simulink library "mylib"  (R2020a)
settings: Solver=VariableStepAuto  StartTime=0.0  StopTime=10.0  RelTol=1e-3
undefined symbols (not defined in the file): d_du_max_pu, dir_to_bus1, dir_to_bus_0L, dir_to_bus_2, dir_to_line1, dir_to_line_0L, dir_to_line_2, du_max_pu, du_ph_max_pu, Fi_0, Fi_T_H, Fi_T_L, Fi_T_M, I0_calc_0L, I0_comp_H, I0_comp_L, I0_comp_M, I0_max_0L, I2_max_2, I_diff1, I_diff2, I_diff3, I_diff4, I_diff5, I_diff_to, I_hight_CT1_G, I_hight_CT2_G, I_low_CT1, I_low_CT2, I_max1, I_max2, I_max3, I_max4, I_max5, I_min_sec_CT1, I_min_sec_CT2, I_unb, Iph_max_0L, Iph_max_2, jmp_in_zone, jmp_in_zone_0L, jmp_in_zone_2, K_dop, max_min1, only_K1_0L, only_K1_2, only_K2_0L, only_K2_2, only_K3_0L, only_K3_2, P_ctl_0, PQ_Fi_ctl_0, Q_ctl_0, S_set_0, set, set1, T_fast, T_I_ctl, T_off, T_on ... (+15)
libraries: $bdroot x184, powerlib_meascontrol x97
(part 3 of 14)

== system mylib/relative ==
  a_re : Inport
  a_im : Inport  Port=2
  1 : Sum  Inputs=+-
  10 : Product  Inputs=*/  RndMeth=Zero  SaturateOnIntegerOverflow=on
  2 : Sum  Inputs=+-
  3 : MinMax  Function=max  Inputs=2
  4 : RelationalOperator  Operator===  OutDataTypeStr=boolean  RndMeth=Simplest
  5 : RelationalOperator  Operator===  OutDataTypeStr=boolean  RndMeth=Simplest
  6 : Switch  Criteria=u2 > Threshold
  7 : RelationalOperator  Operator===  OutDataTypeStr=boolean  RndMeth=Simplest
  8 : Constant  Value=0
  9 : Constant  Value=0.0000001
  fifo1 : Subsystem
  fifo2 : Subsystem
  module1 : Subsystem
  module2 : Subsystem
  module3 : Subsystem
  Y : Outport
  Y_abs : Outport  Port=2
  up : Outport  Port=3
  down : Outport  Port=4
  wires:
  fifo1/1(y0) -> module2/1(Re), 1/1
  fifo1/5(y4) -> module3/1(Re), 1/2
  fifo2/1(y0) -> module2/2(Im), 2/1
  fifo2/5(y4) -> module3/2(Im), 2/2
  1/1 -> module1/1(Re)
  2/1 -> module1/2(Im)
  3/1 -> 5/1, 7/1, 6/3, 4/2
  module2/1(Module) -> 3/1, 4/1
  module3/1(Module) -> 3/2, 5/2
  7/1 -> 6/2
  8/1 -> 7/2
  9/1 -> 6/1
  5/1 -> down/1
  4/1 -> up/1
  module1/1(Module) -> 10/1, Y_abs/1
  6/1 -> 10/2
  10/1 -> Y/1
  a_im/1 -> fifo2/1(y)
  a_re/1 -> fifo1/1(y)

== system mylib/simpcomp ==
  FAre : Inport
  FAim : Inport  Port=2
  FBre : Inport  Port=3
  FBim : Inport  Port=4
  FCre : Inport  Port=5
  FCim : Inport  Port=6
  1 : Constant  Value=-0.5
  {3..5,9..11,18..23} (12 alike) : Sum
  {2,12..16} (6 alike) : Product
  17 : Constant  Value=0.33333333333
  6 : Constant  Value=0.8660254037844386
  7 : Constant  Value=-0.8660254037844386
  orto_MUL_orto : Subsystem
  orto_MUL_orto1 : Subsystem
  orto_MUL_orto2 : Subsystem
  orto_MUL_orto3 : Subsystem
  F0re : Outport
  F0im : Outport  Port=2
  F1re : Outport  Port=3
  F1im : Outport  Port=4
  F2re : Outport  Port=5
  F2im : Outport  Port=6
  wires:
  1/1 -> orto_MUL_orto1/3(F2re), orto_MUL_orto/3(F2re), orto_MUL_orto2/3(F2re), orto_MUL_orto3/3(F2re)
  6/1 -> orto_MUL_orto2/4(F2im), orto_MUL_orto/4(F2im)
  7/1 -> orto_MUL_orto3/4(F2im), orto_MUL_orto1/4(F2im)
  15/1 -> F2im/1
  14/1 -> F2re/1
  16/1 -> F1im/1
  13/1 -> F1re/1
  2/1 -> F0re/1
  12/1 -> F0im/1
  5/1 -> 2/1
  3/1 -> 12/1
  4/1 -> 13/1
  11/1 -> 16/1
  9/1 -> 14/1
  10/1 -> 15/1
  20/1 -> 10/2
  23/1 -> 9/2
  21/1 -> 11/2
  22/1 -> 4/2
  18/1 -> 3/1
  19/1 -> 5/1
  FAim/1 -> 10/1, 3/2, 11/1
  FAre/1 -> 9/1, 5/2, 4/1
  orto_MUL_orto2/2(Fim) -> 20/2
  orto_MUL_orto1/2(Fim) -> 20/1
  orto_MUL_orto2/1(Fre) -> 23/2
  orto_MUL_orto1/1(Fre) -> 23/1
  orto_MUL_orto3/2(Fim) -> 21/2
  orto_MUL_orto/2(Fim) -> 21/1
  orto_MUL_orto3/1(Fre) -> 22/2
  orto_MUL_orto/1(Fre) -> 22/1
  FBre/1 -> orto_MUL_orto1/1(F1re), 19/1, orto_MUL_orto/1(F1re)
  FBim/1 -> orto_MUL_orto1/2(F1im), 18/1, orto_MUL_orto/2(F1im)
  FCim/1 -> 18/2, orto_MUL_orto2/2(F1im), orto_MUL_orto3/2(F1im)
  FCre/1 -> orto_MUL_orto3/1(F1re), 19/2, orto_MUL_orto2/1(F1re)
  17/1 -> 15/2, 14/2, 13/2, 12/2, 2/2, 16/2

== system mylib/st_inverse ==
  block1 : Inport
  block2 : Inport  Port=2
  block3 : Inport  Port=3
  block4 : Inport  Port=4
  in : Inport  Port=5
  alt_in : Inport  Port=6
  jmp : Inport  Port=7
  I_re : Inport  Port=8
  I_im : Inport  Port=9
  1 : Logic  Operator=OR  Inputs=4  AllPortsSameDT=off  OutDataTypeStr=boolean
  Cast To Double : DataTypeConversion  OutDataTypeStr=double
  Constant4 : Constant  Value=jmp_in_zone
  Inverse time-delay : Subsystem  mask{Itd=[14.7, 1, 1], IEC=[4, 3, 9, 0.05], IEC_idr=[4, 7, 2], ANSI=[7, 3, 7, 9.3, 0.08], ANSI_idr=[7, 5, 4.1, 0]}
      mask prompts: Itd "Itd [Ip, Type_ITD, IDR]"; IEC "IEC [IEC_N, ku_IEC, au_IEC, Tb]"; IEC_idr "IEC_idr [IEC_N_idr, ku_IEC_idr, au_IEC_idr]"; ANSI "ANSI [ANSI_N, Au_ANSI, Bu_ANSI, Cu_ANSI, D]"; ANSI_idr "ANSI_idr [ANSI_N_idr, Au_ANSI_idr, Bu_ANSI_idr, Cu_ANSI_idr]"
      mask init: same as mylib/Inverse time-delay
      mask DialogControl Control2 Prompt: Inverse time-delay
      mask DialogControl Control3 Prompt: IEC
      mask DialogControl Control4 Prompt: IEC_idr
      mask DialogControl Control5 Prompt: ANSI
      mask DialogControl Control6 Prompt: ANSI_idr
  Logical Operator14 : Logic  Operator=OR  AllPortsSameDT=off  OutDataTypeStr=boolean
  Logical Operator2 : Logic  AllPortsSameDT=off  OutDataTypeStr=boolean
  Logical Operator3 : Logic  Operator=NOT  AllPortsSameDT=off  OutDataTypeStr=boolean
  Logical Operator8 : Logic  AllPortsSameDT=off  OutDataTypeStr=boolean
  ORTOTOMODULE : $bdroot/ORTOTOMODULE  SystemSampleTime=-1  Latency=0  AutoFrameSizeCalculation=off
  R_TRIG : $bdroot/R_TRIG  SystemSampleTime=-1  Latency=0  AutoFrameSizeCalculation=off
  Variable Transport Delay : VariableTransportDelay  VariableDelayType=Variable transport delay  MaximumDelay=100
  in_1 : Subsystem  mask{in_jmp=[T_reset]}
      mask prompts: in_jmp "in_jmp[T_reset]"
  out_a : $bdroot/out3  out=[T_out]
  avar : Outport
  Y : Outport  Port=2
  fast : Outport  Port=3
  wires:
  block1/1 -> 1/1
  block2/1 -> 1/2
  block3/1 -> 1/3
  block4/1 -> 1/4
  in/1 -> Logical Operator8/2, in_1/2(in)
  R_TRIG/1 -> avar/1
  Constant4/1 -> in_1/1(jmp_in_zone)
  jmp/1 -> in_1/3(jmp)
  Logical Operator3/1 -> Logical Operator2/1
  in_1/1(Y) -> Logical Operator2/2  "Ya"
  1/1 -> Logical Operator3/1
  out_a/1 -> R_TRIG/1, Y/1  "Y_c"
  Logical Operator8/1 -> out_a/1
  Variable Transport Delay/1 -> Logical Operator8/1
  Logical Operator2/1 -> fast/1, Logical Operator14/1
  alt_in/1 -> Logical Operator14/2
  I_im/1 -> ORTOTOMODULE/2
  I_re/1 -> ORTOTOMODULE/1
  ORTOTOMODULE/1 -> Inverse time-delay/1(I)
  Inverse time-delay/1(tp) -> Variable Transport Delay/2
  Inverse time-delay/2(td) -> in_1/4(T_reset)
  Logical Operator14/1 -> Cast To Double/1
  Cast To Double/1 -> Variable Transport Delay/1

== system mylib/tzop_st_v1 ==
  fast1_time : Inport
  fast2_time : Inport  Port=2
  fast3_time : Inport  Port=3
  fast4_time : Inport  Port=4
  fast1_zero : Inport  Port=5
  fast2_zero : Inport  Port=6
  fast3_zero : Inport  Port=7
  fast4_zero : Inport  Port=8
  block1 : Inport  Port=9
  block2 : Inport  Port=10
  block3 : Inport  Port=11
  block4 : Inport  Port=12
  no_dir1 : Inport  Port=13
  no_dir2 : Inport  Port=14
  no_dir3 : Inport  Port=15
  no_dir4 : Inport  Port=16
  dir_to_line : Inport  Port=17
  Ia_re : Inport  Port=18
  Ia_im : Inport  Port=19
  Ib_re : Inport  Port=20
  Ib_im : Inport  Port=21
  Ic_re : Inport  Port=22
  Ic_im : Inport  Port=23
  jmp_a : Inport  Port=24
  jmp_b : Inport  Port=25
  jmp_c : Inport  Port=26
  {1..3,33} (4 alike) : Logic  Operator=OR  Inputs=4  AllPortsSameDT=off  OutDataTypeStr=boolean
  200_det18_ph : Subsystem  mask{det=[0, Iph_max, 0, 0]}
      mask prompts: det "det [max_min, set, dir_to_line, dir_to_bus]"
      mask init:
      | max_min = det(1);
      | set = det(2);
      | dir_to_line = det(3);
      | dir_to_bus = det(4);
  218_det18 : Subsystem  mask{det=[0, I2_max, dir_to_line, dir_to_bus]}
      mask prompts: det "det [max_min, set, dir_to_line, dir_to_bus]"
      mask init:
      | max_min = det(1);
      | set = det(2);
      | dir_to_line = det(3);
      | dir_to_bus = det(4);
  230_st18_ph : Subsystem  AncestorBlock=mylib/230_st18_ph  mask{st18_ph=[only_K1, only_K2, only_K3, jmp_in_zone, T_reset, T_fast, T_st, T_out]}
      mask prompts: st18_ph "st18_ph [only_K1, only_K2, only_K3, jmp_in_zone, T_reset, T_fast, T_st, T_out]"
      mask init:
      | only_K1 = st18_ph(1);
      | only_K2 = st18_ph(2); 
      | only_K3 = st18_ph(3); 
      | jmp_in_zone = st18_ph(4);
      | T_reset = st18_ph(5);
      | T_fast = st18_ph(6); 
      | T_st = st18_ph(7); 
      | T_out = st18_ph(8);
  Constant : Constant
  Constant10 : Constant  Value=0
  Constant11 : Constant  Value=0
  Constant12 : Constant
  Constant13 : Constant  Value=0
  simpcomp : $bdroot/simpcomp  SystemSampleTime=-1  Latency=0  AutoFrameSizeCalculation=off
  avar : Outport
  avar1 : Outport  Port=2
  Y : Outport  Port=3
  Y_a : Outport  Port=4
  Y_b : Outport  Port=5
  Y_c : Outport  Port=6
  fast : Outport  Port=7
  fast_a : Outport  Port=8
  fast_b : Outport  Port=9
  fast_c : Outport  Port=10
  wires:
  Constant13/1 -> 200_det18_ph/2(start2), 200_det18_ph/3(start3), 200_det18_ph/4(start4), 200_det18_ph/6(block2), 200_det18_ph/7(block3), 200_det18_ph/11(no_dir3), 200_det18_ph/12(no_dir4), 200_det18_ph/13(block_a), 200_det18_ph/14(block_b), 200_det18_ph/15(block_c), 200_det18_ph/22(dir_to_line_a), 200_det18_ph/23(dir_to_line_b), 200_det18_ph/24(dir_to_line_c), 200_det18_ph/10(no_dir2), 200_det18_ph/8(block4)
  Constant12/1 -> 200_det18_ph/9(no_dir1)
  1/1 -> 230_st18_ph/3(fast1_zero)
  33/1 -> 230_st18_ph/1(fast1_time)
  218_det18/2(Y) -> 200_det18_ph/1(start1)
  jmp_c/1 -> 230_st18_ph/17(jmp_c)
  jmp_b/1 -> 230_st18_ph/16(jmp_b)
  jmp_a/1 -> 230_st18_ph/15(jmp_a)
  Constant11/1 -> 230_st18_ph/2(fast2_time), 230_st18_ph/4(fast2_zero), 230_st18_ph/6(block2), 230_st18_ph/7(block3), 230_st18_ph/8(block4), 230_st18_ph/12(alt_in_a), 230_st18_ph/13(alt_in_b), 230_st18_ph/14(alt_in_c)
  200_det18_ph/5(Y_c) -> 230_st18_ph/11(in_c)
  200_det18_ph/4(Y_b) -> 230_st18_ph/10(in_b)
  200_det18_ph/3(Y_a) -> 230_st18_ph/9(in_a)
  230_st18_ph/6(fast) -> fast/1
  230_st18_ph/7(fast_a) -> fast_a/1
  230_st18_ph/8(fast_b) -> fast_b/1
  230_st18_ph/9(fast_c) -> fast_c/1
  230_st18_ph/5(Y_c) -> Y_c/1
  230_st18_ph/4(Y_b) -> Y_b/1
  230_st18_ph/3(Y_a) -> Y_a/1
  230_st18_ph/2(Y) -> Y/1
  230_st18_ph/1(avar) -> avar1/1
  2/1 -> 230_st18_ph/5(block1), 218_det18/5(block1)
  3/1 -> 218_det18/9(no_dir1)
  Constant10/1 -> 218_det18/2(start2), 218_det18/3(start3), 218_det18/4(start4), 218_det18/6(block2), 218_det18/7(block3), 218_det18/8(block4), 218_det18/10(no_dir2), 218_det18/11(no_dir3), 218_det18/12(no_dir4)
  Constant/1 -> 218_det18/1(start1)
  dir_to_line/1 -> 218_det18/15(dir_to_line)
  simpcomp/6 -> 218_det18/14(in_im)
  simpcomp/5 -> 218_det18/13(in_re)
  Ic_im/1 -> simpcomp/6, 200_det18_ph/21(in_c_im)
  Ic_re/1 -> simpcomp/5, 200_det18_ph/20(in_c_re)
  Ib_im/1 -> simpcomp/4, 200_det18_ph/19(in_b_im)
  Ib_re/1 -> simpcomp/3, 200_det18_ph/18(in_b_re)
  Ia_im/1 -> simpcomp/2, 200_det18_ph/17(in_a_im)
  Ia_re/1 -> simpcomp/1, 200_det18_ph/16(in_a_re)
  no_dir1/1 -> 3/1
  no_dir3/1 -> 3/3
  no_dir4/1 -> 3/4
  no_dir2/1 -> 3/2
  fast1_time/1 -> 33/1
  fast2_time/1 -> 33/2
  fast3_time/1 -> 33/3
  fast4_time/1 -> 33/4
  fast1_zero/1 -> 1/1
  fast2_zero/1 -> 1/2
  fast3_zero/1 -> 1/3
  fast4_zero/1 -> 1/4
  block1/1 -> 2/1
  block2/1 -> 2/2
  block3/1 -> 2/3
  block4/1 -> 2/4
  218_det18/1(avar) -> avar/1

== system mylib/vect_to_pu ==
  In_re : Inport
  In_im : Inport  Port=2
  1 : Product  Inputs=**
  2 : Sum
  3 : Product  Inputs=*/
  4 : Sqrt  SaturateOnIntegerOverflow=on
  5 : Product  Inputs=**
  6 : Product  Inputs=*/
  out_re : Outport
  out_im : Outport  Port=2
  wires:
  5/1 -> 2/2
  1/1 -> 2/1
  2/1 -> 4/1
  6/1 -> out_re/1
  In_re/1 -> 6/1, 1/2, 1/1
  In_im/1 -> 3/1, 5/2, 5/1
  3/1 -> out_im/1
  4/1 -> 3/2, 6/2

== system mylib/205_st18/Subsystem ==
  T_fast_time : Inport
  T_fast_zero : Inport  Port=2
  "In1 " : Inport  Port=3
  5 : Switch  Criteria=u2 > Threshold
  7 : Switch  Criteria=u2 > Threshold
  T3 : powerlib_meascontrol/Logic/On Delay  DelayType=On delay  delay=T_st  ic=0  Ts=0
  T6 : powerlib_meascontrol/Logic/On Delay  DelayType=On delay  delay=T_fast  ic=0  Ts=0
  T7 : powerlib_meascontrol/Logic/On Delay  DelayType=Off delay  delay=T_fast  ic=0  Ts=0
  Out1 : Outport
  wires:
  "In1 "/1 -> T6/1, 5/1, T3/1
  T7/1 -> 7/2
  T_fast_time/1 -> T7/1
  T6/1 -> 7/1
  T3/1 -> 7/3
  T_fast_zero/1 -> 5/2
  7/1 -> 5/3
  5/1 -> Out1/1

== system mylib/205_st18/in_1 ==
  jmp_in_zone : Inport
  in : Inport  Port=2
  jmp : Inport  Port=3
  1 : Switch  Criteria=u2 > Threshold
  10 : Logic  AllPortsSameDT=off  OutDataTypeStr=boolean
  11 : Logic  Operator=NOT  AllPortsSameDT=off  OutDataTypeStr=boolean
  12 : Memory
  3 : Logic  AllPortsSameDT=off  OutDataTypeStr=boolean
  RS : $bdroot/RS  SystemSampleTime=-1  Latency=0  AutoFrameSizeCalculation=off
  R_TRIG : $bdroot/R_TRIG  SystemSampleTime=-1  Latency=0  AutoFrameSizeCalculation=off
  T1 : powerlib_meascontrol/Logic/On Delay  DelayType=Off delay  delay=T_reset  ic=0  Ts=0
  T2 : powerlib_meascontrol/Logic/On Delay  DelayType=On delay  delay=T_reset  ic=0  Ts=0
  Y : Outport
  wires:
  RS/1 -> 12/1, Y/1
  in/1 -> 11/1, R_TRIG/1, 1/3
  R_TRIG/1 -> 1/1
  jmp_in_zone/1 -> 1/2
  11/1 -> 10/2
  10/1 -> T2/1
  T1/1 -> 3/2
  1/1 -> 3/1
  jmp/1 -> T1/1
  12/1 -> 10/1
  T2/1 -> RS/2
  3/1 -> RS/1

== system mylib/219_onm_v1/onm_fi_v1 ==
  U_re : Inport
  U_im : Inport  Port=2
  I_re : Inport  Port=3
  I_im : Inport  Port=4
  Constant : Constant  Value=-1
  Constant1 : Constant  Value=-1
  Constant2 : Constant  Value=S_set
  Constant3 : Constant  Value=Fi
  Constant4 : Constant  Value=0.0174532925
  Constant5 : Constant  Value=-1
  Cos : Trigonometry  Operator=cos
  Divide{,1..3} (4 alike) : Product  Inputs=**
  Logical Operator : Logic  Operator=NOT  AllPortsSameDT=off  OutDataTypeStr=boolean
  Logical Operator1 : Logic  Operator=NOT  AllPortsSameDT=off  OutDataTypeStr=boolean
  Relational Operator : RelationalOperator  Operator=<  OutDataTypeStr=boolean  RndMeth=Simplest
  Relational Operator1 : RelationalOperator  Operator=>  OutDataTypeStr=boolean  RndMeth=Simplest
  S_calc : $bdroot/orto_MUL_orto  SystemSampleTime=-1  Latency=0  AutoFrameSizeCalculation=off
  S_protection_calc : $bdroot/orto_MUL_orto  SystemSampleTime=-1  Latency=0  AutoFrameSizeCalculation=off
  Sin : Trigonometry
  Switch : Switch  Criteria=u2 > Threshold
  Y : Outport
  wires:
  Relational Operator1/1 -> Logical Operator/1, Switch/3
  Logical Operator/1 -> Switch/2
  Logical Operator1/1 -> Switch/1
  Switch/1 -> Y/1
  Relational Operator/1 -> Logical Operator1/1
  S_protection_calc/1 -> Relational Operator/1, Relational Operator1/1
  Constant2/1 -> Divide3/1, Relational Operator1/2
  Constant5/1 -> Divide3/2
  Divide3/1 -> Relational Operator/2
  Divide1/1 -> S_protection_calc/4
  Cos/1 -> S_protection_calc/3
  Constant3/1 -> Divide2/1
  Constant4/1 -> Divide2/2
  Divide2/1 -> Cos/1, Sin/1
  Constant1/1 -> Divide1/2
  Sin/1 -> Divide1/1
  S_calc/2 -> S_protection_calc/2
  S_calc/1 -> S_protection_calc/1
  Constant/1 -> Divide/2
  Divide/1 -> S_calc/4
  I_im/1 -> Divide/1
  I_re/1 -> S_calc/3
  U_re/1 -> S_calc/1
  U_im/1 -> S_calc/2

== system mylib/219_onm_v1/pq_dir_v1 ==
  U_re : Inport
  U_im : Inport  Port=2
  I_re : Inport  Port=3
  I_im : Inport  Port=4
  max_comp : Inport  Port=5
  Add : Sum
  Constant : Constant  Value=-1
  Constant1 : Constant  Value=-1
  Constant2 : Constant  Value=P_ctl
  Constant3 : Constant  Value=Q_ctl
  Constant4 : Constant  Value=0
  Constant5 : Constant  Value=0
  Divide{,1..3} (4 alike) : Product  Inputs=**
  Logical Operator : Logic  Operator=NOT  AllPortsSameDT=off  OutDataTypeStr=boolean
  Logical Operator1 : Logic  AllPortsSameDT=off  OutDataTypeStr=boolean
  Logical Operator2 : Logic  AllPortsSameDT=off  OutDataTypeStr=boolean
  Logical Operator3 : Logic  Operator=OR  AllPortsSameDT=off  OutDataTypeStr=boolean
  Relational Operator1 : RelationalOperator  Operator=>  OutDataTypeStr=boolean  RndMeth=Simplest
  Relational Operator2 : RelationalOperator  Operator=>  OutDataTypeStr=boolean  RndMeth=Simplest
  Relational Operator3 : RelationalOperator  Operator=>  OutDataTypeStr=boolean  RndMeth=Simplest
  S_calc : $bdroot/orto_MUL_orto  SystemSampleTime=-1  Latency=0  AutoFrameSizeCalculation=off
  Switch : Switch  Criteria=u2 > Threshold
  Switch1 : Switch  Criteria=u2 > Threshold
  Y : Outport
  wires:
  Relational Operator1/1 -> Logical Operator1/1
  Relational Operator2/1 -> Logical Operator2/1
  Switch/1 -> Logical Operator1/2
  Switch1/1 -> Logical Operator2/2
  Logical Operator3/1 -> Y/1
  Logical Operator2/1 -> Logical Operator3/2
  Logical Operator1/1 -> Logical Operator3/1
  Constant3/1 -> Switch1/3
  Relational Operator3/1 -> Switch/1, Logical Operator/1
  Logical Operator/1 -> Switch1/1
  Constant2/1 -> Switch/3
  max_comp/1 -> Switch/2, Switch1/2
  Add/1 -> Relational Operator3/1
  Constant5/1 -> Relational Operator3/2
  Divide1/1 -> Add/2
  Divide2/1 -> Add/1
  Constant1/1 -> Divide3/2
  Divide3/1 -> Divide1/2
  Constant4/1 -> Relational Operator1/2, Relational Operator2/2
  S_calc/2 -> Relational Operator2/1, Divide1/1, Divide3/1
  S_calc/1 -> Relational Operator1/1, Divide2/1, Divide2/2
  Constant/1 -> Divide/2
  Divide/1 -> S_calc/4
  I_im/1 -> Divide/1
  I_re/1 -> S_calc/3
  U_re/1 -> S_calc/1
  U_im/1 -> S_calc/2

== system mylib/230_st18_ph/Subsystem ==
  T_fast_time : Inport
  T_fast_zero : Inport  Port=2
  "In1 " : Inport  Port=3
  "In2 " : Inport  Port=4
  "In3 " : Inport  Port=5
  {1..5,7} (6 alike) : Switch  Criteria=u2 > Threshold
  T1 : powerlib_meascontrol/Logic/On Delay  DelayType=On delay  delay=T_st  ic=0  Ts=0
  T2 : powerlib_meascontrol/Logic/On Delay  DelayType=On delay  delay=T_st  ic=0  Ts=0
  T3 : powerlib_meascontrol/Logic/On Delay  DelayType=On delay  delay=T_st  ic=0  Ts=0
  T4 : powerlib_meascontrol/Logic/On Delay  DelayType=On delay  delay=T_fast  ic=0  Ts=0
  T5 : powerlib_meascontrol/Logic/On Delay  DelayType=On delay  delay=T_fast  ic=0  Ts=0
  T6 : powerlib_meascontrol/Logic/On Delay  DelayType=On delay  delay=T_fast  ic=0  Ts=0
  T7 : powerlib_meascontrol/Logic/On Delay  DelayType=Off delay  delay=T_fast  ic=0  Ts=0
  Out1 : Outport
  Out2 : Outport  Port=2
  Out3 : Outport  Port=3
  wires:
  "In3 "/1 -> T4/1, T2/1, 4/1
  "In2 "/1 -> 3/1, T5/1, T1/1
  "In1 "/1 -> 5/1, T3/1, T6/1
  T7/1 -> 2/2, 1/2, 7/2
  T_fast_time/1 -> T7/1
  T4/1 -> 2/1
  T5/1 -> 1/1
  T6/1 -> 7/1
  T3/1 -> 7/3
  T1/1 -> 1/3
  T2/1 -> 2/3
  T_fast_zero/1 -> 5/2, 3/2, 4/2
  7/1 -> 5/3
  1/1 -> 3/3
  2/1 -> 4/3
  5/1 -> Out1/1
  3/1 -> Out2/1
  4/1 -> Out3/1

== system mylib/230_st18_ph/in_1 ==
  jmp_in_zone : Inport
  in : Inport  Port=2
  jmp : Inport  Port=3
  1 : Switch  Criteria=u2 > Threshold
  10 : Logic  AllPortsSameDT=off  OutDataTypeStr=boolean
  11 : Logic  Operator=NOT  AllPortsSameDT=off  OutDataTypeStr=boolean
  12 : Memory
  3 : Logic  AllPortsSameDT=off  OutDataTypeStr=boolean
  RS : $bdroot/RS  SystemSampleTime=-1  Latency=0  AutoFrameSizeCalculation=off
  R_TRIG : $bdroot/R_TRIG  SystemSampleTime=-1  Latency=0  AutoFrameSizeCalculation=off
  T1 : powerlib_meascontrol/Logic/On Delay  DelayType=Off delay  delay=T_reset  ic=0  Ts=0
  T2 : powerlib_meascontrol/Logic/On Delay  DelayType=On delay  delay=T_reset  ic=0  Ts=0
  Y : Outport
  wires:
  RS/1 -> 12/1, Y/1
  in/1 -> 11/1, R_TRIG/1, 1/3
  R_TRIG/1 -> 1/1
  jmp_in_zone/1 -> 1/2
  11/1 -> 10/2
  10/1 -> T2/1
  T1/1 -> 3/2
  1/1 -> 3/1
  jmp/1 -> T1/1
  12/1 -> 10/1
  T2/1 -> RS/2
  3/1 -> RS/1

== system mylib/230_st18_ph/in_2 ==
  jmp_in_zone : Inport
  in : Inport  Port=2
  jmp : Inport  Port=3
  1 : Switch  Criteria=u2 > Threshold
  10 : Logic  AllPortsSameDT=off  OutDataTypeStr=boolean
  11 : Logic  Operator=NOT  AllPortsSameDT=off  OutDataTypeStr=boolean
  12 : Memory
  3 : Logic  AllPortsSameDT=off  OutDataTypeStr=boolean
  RS : $bdroot/RS  SystemSampleTime=-1  Latency=0  AutoFrameSizeCalculation=off
  R_TRIG : $bdroot/R_TRIG  SystemSampleTime=-1  Latency=0  AutoFrameSizeCalculation=off
  T1 : powerlib_meascontrol/Logic/On Delay  DelayType=Off delay  delay=T_reset  ic=0  Ts=0
  T2 : powerlib_meascontrol/Logic/On Delay  DelayType=On delay  delay=T_reset  ic=0  Ts=0
  Y : Outport
  wires:
  RS/1 -> 12/1, Y/1
  in/1 -> 11/1, R_TRIG/1, 1/3
  R_TRIG/1 -> 1/1
  jmp_in_zone/1 -> 1/2
  11/1 -> 10/2
  10/1 -> T2/1
  T1/1 -> 3/2
  1/1 -> 3/1
  jmp/1 -> T1/1
  12/1 -> 10/1
  T2/1 -> RS/2
  3/1 -> RS/1

== system mylib/230_st18_ph/in_3 ==
  jmp_in_zone : Inport
  in : Inport  Port=2
  jmp : Inport  Port=3
  1 : Switch  Criteria=u2 > Threshold
  10 : Logic  AllPortsSameDT=off  OutDataTypeStr=boolean
  11 : Logic  Operator=NOT  AllPortsSameDT=off  OutDataTypeStr=boolean
  12 : Memory
  3 : Logic  AllPortsSameDT=off  OutDataTypeStr=boolean
  RS : $bdroot/RS  SystemSampleTime=-1  Latency=0  AutoFrameSizeCalculation=off
  R_TRIG : $bdroot/R_TRIG  SystemSampleTime=-1  Latency=0  AutoFrameSizeCalculation=off
  T1 : powerlib_meascontrol/Logic/On Delay  DelayType=Off delay  delay=T_reset  ic=0  Ts=0
  T2 : powerlib_meascontrol/Logic/On Delay  DelayType=On delay  delay=T_reset  ic=0  Ts=0
  Y : Outport
  wires:
  RS/1 -> 12/1, Y/1
  in/1 -> 11/1, R_TRIG/1, 1/3
  R_TRIG/1 -> 1/1
  jmp_in_zone/1 -> 1/2
  11/1 -> 10/2
  10/1 -> T2/1
  T1/1 -> 3/2
  1/1 -> 3/1
  jmp/1 -> T1/1
  12/1 -> 10/1
  T2/1 -> RS/2
  3/1 -> RS/1

== system mylib/230_st18_ph/k_type ==
  In_a : Inport
  In_b : Inport  Port=2
  In_ c : Inport  Port=3
  only_K1 : Inport  Port=4
  only_K2 : Inport  Port=5
  only_K3 : Inport  Port=6
  1 : Switch  Criteria=u2 > Threshold
  Logical Operator{1,12,18..27} (12 alike) : Logic  Operator=NOT  AllPortsSameDT=off  OutDataTypeStr=boolean
  Logical Operator10 : Logic  AllPortsSameDT=off  OutDataTypeStr=boolean
  Logical Operator{2..4,7..8,11,14,17} (8 alike) : Logic  Inputs=3  AllPortsSameDT=off  OutDataTypeStr=boolean
  Logical Operator{5..6,13,16} (4 alike) : Logic  Operator=OR  Inputs=3  AllPortsSameDT=off  OutDataTypeStr=boolean
  Logical Operator15 : Logic  AllPortsSameDT=off  OutDataTypeStr=boolean
  Logical Operator9 : Logic  AllPortsSameDT=off  OutDataTypeStr=boolean
  out : Outport
  wires:
  Logical Operator12/1 -> Logical Operator11/2
  Logical Operator1/1 -> Logical Operator11/3
  Logical Operator2/1 -> Logical Operator5/2
  Logical Operator11/1 -> Logical Operator5/1
  Logical Operator3/1 -> Logical Operator5/3
  Logical Operator4/1 -> Logical Operator6/1
  Logical Operator7/1 -> Logical Operator6/2
  Logical Operator8/1 -> Logical Operator6/3
  Logical Operator5/1 -> Logical Operator9/2
  Logical Operator6/1 -> Logical Operator10/2
  Logical Operator9/1 -> Logical Operator13/1
  Logical Operator10/1 -> Logical Operator13/2
  Logical Operator15/1 -> Logical Operator13/3
  Logical Operator14/1 -> Logical Operator15/2
  Logical Operator19/1 -> Logical Operator17/1
  Logical Operator18/1 -> Logical Operator17/2
  Logical Operator20/1 -> Logical Operator17/3
  Logical Operator21/1 -> Logical Operator8/3
  Logical Operator22/1 -> Logical Operator7/2
  Logical Operator23/1 -> Logical Operator4/1
  Logical Operator24/1 -> Logical Operator2/1
  In_a/1 -> Logical Operator26/1, Logical Operator23/1, Logical Operator7/1, Logical Operator8/1, Logical Operator16/1, Logical Operator14/1, Logical Operator24/1, Logical Operator11/1
  Logical Operator25/1 -> Logical Operator2/3
  Logical Operator26/1 -> Logical Operator3/1
  Logical Operator27/1 -> Logical Operator3/2
  In_b/1 -> Logical Operator12/1, Logical Operator2/2, Logical Operator27/1, Logical Operator4/2, Logical Operator22/1, Logical Operator8/2, Logical Operator16/2, Logical Operator14/2
  only_K1/1 -> Logical Operator19/1, Logical Operator9/1
  only_K2/1 -> Logical Operator18/1, Logical Operator10/1
  only_K3/1 -> Logical Operator15/1, Logical Operator20/1
  Logical Operator17/1 -> 1/2
  1/1 -> out/1
  Logical Operator13/1 -> 1/3
  Logical Operator16/1 -> 1/1
  In_ c/1 -> Logical Operator1/1, Logical Operator25/1, Logical Operator3/3, Logical Operator4/3, Logical Operator7/3, Logical Operator21/1, Logical Operator16/3, Logical Operator14/3

== system mylib/231_u_block_v1/RS ==
  S : Inport
  R : Inport  Port=2
  12 : Logic  AllPortsSameDT=off  OutDataTypeStr=boolean
  13 : Logic  Operator=NOT  AllPortsSameDT=off  OutDataTypeStr=boolean
  14 : Memory
  15 : Logic  Operator=OR  AllPortsSameDT=off  OutDataTypeStr=boolean
  Q : Outport
  wires:
  13/1 -> 12/2
  S/1 -> 15/2
  R/1 -> 13/1
  15/1 -> 12/1
  12/1 -> Q/1, 14/1
  14/1 -> 15/1

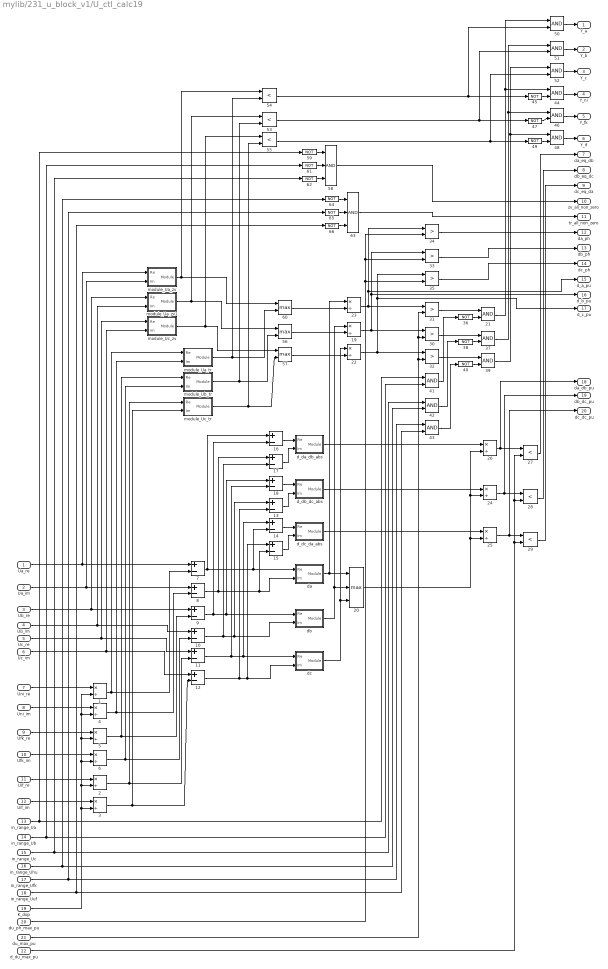
== system mylib/231_u_block_v1/U_ctl_calc19 ==
  Ua_re : Inport
  Ua_im : Inport  Port=2
  Ub_re : Inport  Port=3
  Ub_im : Inport  Port=4
  Uc_re : Inport  Port=5
  Uc_im : Inport  Port=6
  Uni_re : Inport  Port=7
  Uni_im : Inport  Port=8
  Ufk_re : Inport  Port=9
  Ufk_im : Inport  Port=10
  Uif_re : Inport  Port=11
  Uif_im : Inport  Port=12
  in_range_Ua : Inport  Port=13
  in_range_Ub : Inport  Port=14
  in_range_Uc : Inport  Port=15
  in_range_Uhu : Inport  Port=16
  in_range_Ufk : Inport  Port=17
  in_range_Uuf : Inport  Port=18
  K_dop : Inport  Port=19
  du_ph_max_pu : Inport  Port=20
  du_max_pu : Inport  Port=21
  d_du_max_pu : Inport  Port=22
  {1..6,19,22..26} (12 alike) : Product  Inputs=*/  RndMeth=Zero  SaturateOnIntegerOverflow=on
  {7..18} (12 alike) : Sum  Inputs=+-
  20 : MinMax  Function=max  Inputs=3
  {21,37,39,41..44,46,48,50..52} (12 alike) : Logic  AllPortsSameDT=off  OutDataTypeStr=boolean
  {27..29,53..55} (6 alike) : RelationalOperator  Operator=<  OutDataTypeStr=boolean  RndMeth=Simplest
  {30..35} (6 alike) : RelationalOperator  Operator=>  OutDataTypeStr=boolean  RndMeth=Simplest
  {36,38,40,45,47,49,59,61..62,64..66} (12 alike) : Logic  Operator=NOT  AllPortsSameDT=off  OutDataTypeStr=boolean
  56 : MinMax  Function=max  Inputs=2
  57 : MinMax  Function=max  Inputs=2
  58 : Logic  Inputs=3  AllPortsSameDT=off  OutDataTypeStr=boolean
  60 : MinMax  Function=max  Inputs=2
  63 : Logic  Inputs=3  AllPortsSameDT=off  OutDataTypeStr=boolean
  d_da_db_abs : Subsystem
  d_db_dc_abs : Subsystem
  d_dc_da_abs : Subsystem
  da : Subsystem
  db : Subsystem
  dc : Subsystem
  module_Ua_tr : Subsystem
  module_Ua_zv : Subsystem
  module_Ua_zv1 : Subsystem
  module_Ub_tr : Subsystem
  module_Uc_tr : Subsystem
  module_Uc_zv : Subsystem
  Y_a : Outport
  Y_b : Outport  Port=2
  Y_c : Outport  Port=3
  Y_ni : Outport  Port=4
  Y_fk : Outport  Port=5
  Y_if : Outport  Port=6
  da_eq_db : Outport  Port=7
  db_eq_dc : Outport  Port=8
  dc_eq_da : Outport  Port=9
  zv_all_non_zero : Outport  Port=10
  tr_all_non_zero : Outport  Port=11
  da_ph : Outport  Port=12
  db_ph : Outport  Port=13
  dc_ph : Outport  Port=14
  d_a_pu : Outport  Port=15
  d_b_pu : Outport  Port=16
  d_c_pu : Outport  Port=17
  da_db_pu : Outport  Port=18
  db_dc_pu : Outport  Port=19
  dc_dc_pu : Outport  Port=20
  wires:
  Uni_re/1 -> 1/1
  Uif_im/1 -> 3/1
  Uif_re/1 -> 2/1
  Ufk_re/1 -> 5/1
  Uni_im/1 -> 4/1
  Ufk_im/1 -> 6/1
  K_dop/1 -> 1/2, 4/2, 5/2, 6/2, 2/2, 3/2
  Ua_re/1 -> module_Ua_zv/1(Re), 7/1
  Ua_im/1 -> module_Ua_zv/2(Im), 8/1
  Ub_re/1 -> module_Ua_zv1/1(Re), 9/1
  Ub_im/1 -> module_Ua_zv1/2(Im), 10/1
  Uc_re/1 -> module_Uc_zv/1(Re), 11/1
  Uc_im/1 -> module_Uc_zv/2(Im), 12/1
  14/1 -> d_dc_da_abs/1(Re)
  15/1 -> d_dc_da_abs/2(Im)
  18/1 -> d_db_dc_abs/1(Re)
  13/1 -> d_db_dc_abs/2(Im)
  16/1 -> d_da_db_abs/1(Re)
  17/1 -> d_da_db_abs/2(Im)
  7/1 -> 16/1, 14/2, da/1(Re)
  9/1 -> 16/2, 18/1, db/1(Re)
  10/1 -> 17/2, 13/1, db/2(Im)
  11/1 -> 18/2, 14/1, dc/1(Re)
  12/1 -> 13/2, 15/1, dc/2(Im)
  dc/1(Module) -> 22/1, 20/3
  db/1(Module) -> 19/1, 20/2
  da/1(Module) -> 23/1, 20/1
  d_da_db_abs/1(Module) -> 26/1
  d_db_dc_abs/1(Module) -> 24/1
  d_dc_da_abs/1(Module) -> 25/1
  20/1 -> 26/2, 24/2, 25/2
  26/1 -> da_db_pu/1, 27/1
  24/1 -> db_dc_pu/1, 28/1
  25/1 -> dc_dc_pu/1, 29/1
  27/1 -> da_eq_db/1
  28/1 -> db_eq_dc/1
  29/1 -> dc_eq_da/1
  22/1 -> d_c_pu/1, 35/1, 32/1
  19/1 -> d_b_pu/1, 33/1, 30/1
  23/1 -> d_a_pu/1, 34/1, 31/1
  du_max_pu/1 -> 31/2, 30/2, 32/2
  36/1 -> 21/2
  38/1 -> 37/2
  40/1 -> 39/2
  31/1 -> 21/1
  30/1 -> 37/1
  32/1 -> 39/1
  41/1 -> 36/1
  42/1 -> 38/1
  43/1 -> 40/1
  in_range_Ub/1 -> 61/1, 41/2
  in_range_Uc/1 -> 62/1, 42/1
  in_range_Uhu/1 -> 64/1, 42/2
  in_range_Ufk/1 -> 65/1, 43/1
  in_range_Uuf/1 -> 66/1, 43/2
  d_du_max_pu/1 -> 29/2, 28/2, 27/2
  du_ph_max_pu/1 -> 35/2, 33/2, 34/2
  34/1 -> da_ph/1
  33/1 -> db_ph/1
  35/1 -> dc_ph/1
  45/1 -> 44/2
  47/1 -> 46/2
  49/1 -> 48/2
  21/1 -> 44/1, 50/1
  37/1 -> 46/1, 51/1
  39/1 -> 48/1, 52/1
  48/1 -> Y_if/1
  46/1 -> Y_fk/1
  44/1 -> Y_ni/1
  52/1 -> Y_c/1
  50/1 -> Y_a/1
  51/1 -> Y_b/1
  55/1 -> 52/2, 49/1
  53/1 -> 51/2, 47/1
  54/1 -> 50/2, 45/1
  57/1 -> 22/2
  56/1 -> 19/2
  60/1 -> 23/2
  module_Uc_tr/1(Module) -> 55/2, 57/2
  module_Ub_tr/1(Module) -> 53/2, 56/2
  module_Ua_tr/1(Module) -> 54/2, 60/2
  module_Uc_zv/1(Module) -> 55/1, 57/1
  module_Ua_zv/1(Module) -> 54/1, 60/1
  module_Ua_zv1/1(Module) -> 53/1, 56/1
  59/1 -> 58/1
  61/1 -> 58/2
  62/1 -> 58/3
  64/1 -> 63/1
  65/1 -> 63/2
  66/1 -> 63/3
  in_range_Ua/1 -> 41/1, 59/1
  63/1 -> tr_all_non_zero/1
  58/1 -> zv_all_non_zero/1
  8/1 -> 17/1, 15/2, da/2(Im)
  1/1 -> module_Ua_tr/1(Re), 7/2
  4/1 -> module_Ua_tr/2(Im), 8/2
  5/1 -> module_Ub_tr/1(Re), 9/2
  6/1 -> module_Ub_tr/2(Im), 10/2
  2/1 -> module_Uc_tr/1(Re), 11/2
  3/1 -> module_Uc_tr/2(Im), 12/2

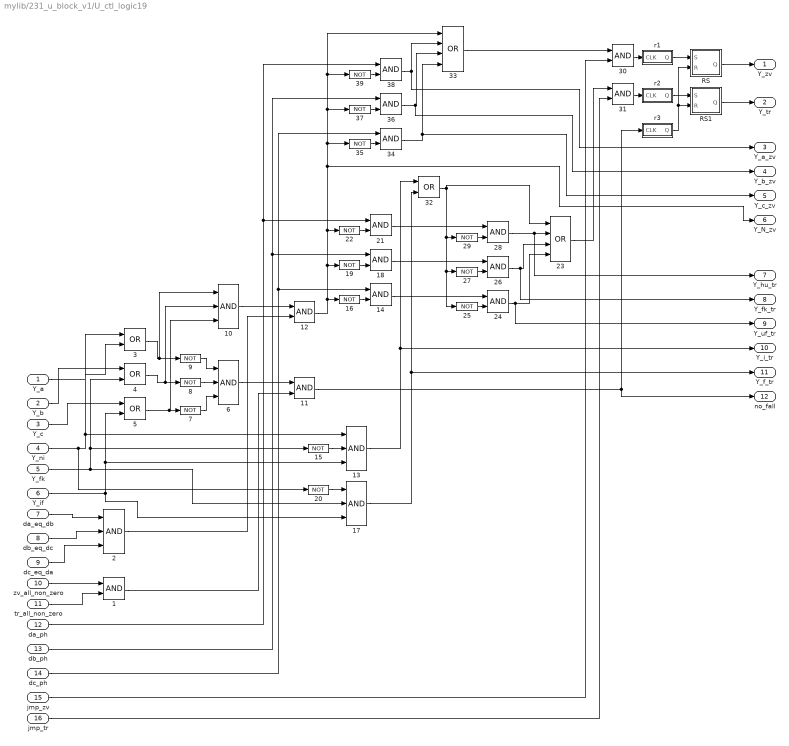
== system mylib/231_u_block_v1/U_ctl_logic19 ==
  Y_a : Inport
  Y_b : Inport  Port=2
  Y_c : Inport  Port=3
  Y_ni : Inport  Port=4
  Y_fk : Inport  Port=5
  Y_if : Inport  Port=6
  da_eq_db : Inport  Port=7
  db_eq_dc : Inport  Port=8
  dc_eq_da : Inport  Port=9
  zv_all_non_zero : Inport  Port=10
  tr_all_non_zero : Inport  Port=11
  da_ph : Inport  Port=12
  db_ph : Inport  Port=13
  dc_ph : Inport  Port=14
  jmp_zv : Inport  Port=15
  jmp_tr : Inport  Port=16
  {1,11..12,14,18,21,24,26,28,30..31,34,36,38} (14 alike) : Logic  AllPortsSameDT=off  OutDataTypeStr=boolean
  {2,6,10,13,17} (5 alike) : Logic  Inputs=3  AllPortsSameDT=off  OutDataTypeStr=boolean
  {7..9,15..16,19..20,22,25,27,29,35,37,39} (14 alike) : Logic  Operator=NOT  AllPortsSameDT=off  OutDataTypeStr=boolean
  23 : Logic  Operator=OR  Inputs=4  AllPortsSameDT=off  OutDataTypeStr=boolean
  {3..5,32} (4 alike) : Logic  Operator=OR  AllPortsSameDT=off  OutDataTypeStr=boolean
  33 : Logic  Operator=OR  Inputs=4  AllPortsSameDT=off  OutDataTypeStr=boolean
  RS : Subsystem
  RS1 : Subsystem
  r1 : Subsystem
  r2 : Subsystem
  r3 : Subsystem
  Y_zv : Outport
  Y_tr : Outport  Port=2
  Y_a_zv : Outport  Port=3
  Y_b_zv : Outport  Port=4
  Y_c_zv : Outport  Port=5
  Y_N_zv : Outport  Port=6
  Y_hu_tr : Outport  Port=7
  Y_fk_tr : Outport  Port=8
  Y_uf_tr : Outport  Port=9
  Y_i_tr : Outport  Port=10
  Y_f_tr : Outport  Port=11
  no_fall : Outport  Port=12
  wires:
  zv_all_non_zero/1 -> 1/1
  tr_all_non_zero/1 -> 1/2
  da_eq_db/1 -> 2/1
  db_eq_dc/1 -> 2/2
  dc_eq_da/1 -> 2/3
  Y_a/1 -> 3/1
  Y_ni/1 -> 3/2, 13/1, 20/1
  Y_b/1 -> 4/1
  Y_fk/1 -> 17/2, 4/2, 15/1
  Y_c/1 -> 5/1
  Y_if/1 -> 13/3, 5/2, 17/3
  5/1 -> 10/3, 7/1
  7/1 -> 6/3
  9/1 -> 6/1
  3/1 -> 10/1, 9/1
  8/1 -> 6/2
  4/1 -> 10/2, 8/1
  6/1 -> 11/1
  1/1 -> 11/2
  10/1 -> 12/1
  2/1 -> 12/2
  15/1 -> 13/2
  20/1 -> 17/1
  16/1 -> 14/2
  19/1 -> 18/2
  22/1 -> 21/2
  12/1 -> 39/1, 33/1, 37/1, 35/1, Y_N_zv/1, 22/1, 19/1, 16/1
  25/1 -> 24/2
  27/1 -> 26/2
  29/1 -> 28/2
  21/1 -> 28/1
  18/1 -> 26/1
  14/1 -> 24/1
  24/1 -> Y_uf_tr/1, 23/4
  26/1 -> Y_fk_tr/1, 23/3
  28/1 -> Y_hu_tr/1, 23/2
  30/1 -> r1/1(CLK)
  r1/1(Q) -> RS/1(S)
  31/1 -> r2/1(CLK)
  r2/1(Q) -> RS1/1(S)
  r3/1(Q) -> RS1/2(R), RS/2(R)
  RS/1(Q) -> Y_zv/1
  RS1/1(Q) -> Y_tr/1
  32/1 -> 23/1, 25/1, 27/1, 29/1
  35/1 -> 34/2
  37/1 -> 36/2
  39/1 -> 38/2
  34/1 -> Y_c_zv/1, 33/4
  38/1 -> Y_a_zv/1, 33/2
  36/1 -> Y_b_zv/1, 33/3
  33/1 -> 30/1
  23/1 -> 31/1
  da_ph/1 -> 38/1, 21/1
  db_ph/1 -> 18/1, 36/1
  dc_ph/1 -> 14/1, 34/1
  jmp_zv/1 -> 30/2
  jmp_tr/1 -> 31/2
  13/1 -> Y_i_tr/1, 32/1
  17/1 -> Y_f_tr/1, 32/2
  11/1 -> no_fall/1, r3/1(CLK)

== system mylib/231_u_block_v1/oscillo1 ==
  CLK : Inport
  26 : Logic  AllPortsSameDT=off  OutDataTypeStr=boolean
  27 : Logic  Operator=NOT  AllPortsSameDT=off  OutDataTypeStr=boolean
  Memory : Memory
  Q : Outport
  wires:
  27/1 -> 26/2
  Memory/1 -> 27/1
  CLK/1 -> Memory/1, 26/1
  26/1 -> Q/1

== system mylib/231_u_block_v1/oscillo2 ==
  CLK : Inport
  26 : Logic  AllPortsSameDT=off  OutDataTypeStr=boolean
  27 : Logic  Operator=NOT  AllPortsSameDT=off  OutDataTypeStr=boolean
  Memory : Memory
  Q : Outport
  wires:
  27/1 -> 26/2
  Memory/1 -> 27/1
  CLK/1 -> Memory/1, 26/1
  26/1 -> Q/1

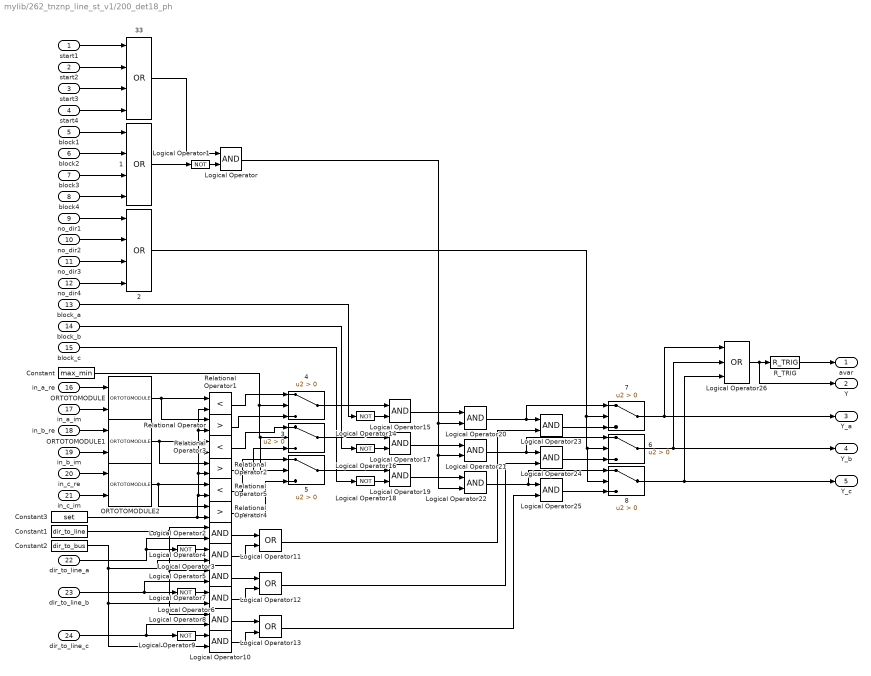
== system mylib/262_tnznp_line_st_v1/200_det18_ph ==
  start1 : Inport
  start2 : Inport  Port=2
  start3 : Inport  Port=3
  start4 : Inport  Port=4
  block1 : Inport  Port=5
  block2 : Inport  Port=6
  block3 : Inport  Port=7
  block4 : Inport  Port=8
  no_dir1 : Inport  Port=9
  no_dir2 : Inport  Port=10
  no_dir3 : Inport  Port=11
  no_dir4 : Inport  Port=12
  block_a : Inport  Port=13
  block_b : Inport  Port=14
  block_c : Inport  Port=15
  in_a_re : Inport  Port=16
  in_a_im : Inport  Port=17
  in_b_re : Inport  Port=18
  in_b_im : Inport  Port=19
  in_c_re : Inport  Port=20
  in_c_im : Inport  Port=21
  dir_to_line_a : Inport  Port=22
  dir_to_line_b : Inport  Port=23
  dir_to_line_c : Inport  Port=24
  1 : Logic  Operator=OR  Inputs=4  AllPortsSameDT=off  OutDataTypeStr=boolean
  2 : Logic  Operator=OR  Inputs=4  AllPortsSameDT=off  OutDataTypeStr=boolean
  {3..8} (6 alike) : Switch  Criteria=u2 > Threshold
  33 : Logic  Operator=OR  Inputs=4  AllPortsSameDT=off  OutDataTypeStr=boolean
  Constant : Constant  Value=max_min
  Constant1 : Constant  Value=dir_to_line
  Constant2 : Constant  Value=dir_to_bus
  Constant3 : Constant  Value=set
  Logical Operator{,2,4..5,7..8,10,15,17,19..25} (16 alike) : Logic  AllPortsSameDT=off  OutDataTypeStr=boolean
  Logical Operator{1,3,6,9,14,16,18} (7 alike) : Logic  Operator=NOT  AllPortsSameDT=off  OutDataTypeStr=boolean
  Logical Operator11 : Logic  Operator=OR  AllPortsSameDT=off  OutDataTypeStr=boolean
  Logical Operator12 : Logic  Operator=OR  AllPortsSameDT=off  OutDataTypeStr=boolean
  Logical Operator13 : Logic  Operator=OR  AllPortsSameDT=off  OutDataTypeStr=boolean
  Logical Operator26 : Logic  Operator=OR  Inputs=3  AllPortsSameDT=off  OutDataTypeStr=boolean
  ORTOTOMODULE : $bdroot/ORTOTOMODULE  SystemSampleTime=-1  Latency=0  AutoFrameSizeCalculation=off
  ORTOTOMODULE1 : $bdroot/ORTOTOMODULE  SystemSampleTime=-1  Latency=0  AutoFrameSizeCalculation=off
  ORTOTOMODULE2 : $bdroot/ORTOTOMODULE  SystemSampleTime=-1  Latency=0  AutoFrameSizeCalculation=off
  R_TRIG : $bdroot/R_TRIG  SystemSampleTime=-1  Latency=0  AutoFrameSizeCalculation=off
  Relational Operator : RelationalOperator  Operator=>  OutDataTypeStr=boolean  RndMeth=Simplest
  Relational Operator1 : RelationalOperator  Operator=<  OutDataTypeStr=boolean  RndMeth=Simplest
  Relational Operator2 : RelationalOperator  Operator=>  OutDataTypeStr=boolean  RndMeth=Simplest
  Relational Operator3 : RelationalOperator  Operator=<  OutDataTypeStr=boolean  RndMeth=Simplest
  Relational Operator4 : RelationalOperator  Operator=>  OutDataTypeStr=boolean  RndMeth=Simplest
  Relational Operator5 : RelationalOperator  Operator=<  OutDataTypeStr=boolean  RndMeth=Simplest
  avar : Outport
  Y : Outport  Port=2
  Y_a : Outport  Port=3
  Y_b : Outport  Port=4
  Y_c : Outport  Port=5
  wires:
  in_b_re/1 -> ORTOTOMODULE1/1
  R_TRIG/1 -> avar/1
  Logical Operator26/1 -> R_TRIG/1, Y/1
  7/1 -> Logical Operator26/1, Y_a/1
  6/1 -> Logical Operator26/2, Y_b/1
  8/1 -> Logical Operator26/3, Y_c/1
  Logical Operator25/1 -> 8/3
  Logical Operator23/1 -> 7/3
  Logical Operator24/1 -> 6/3
  Logical Operator13/1 -> Logical Operator25/2
  2/1 -> 7/2, 6/2, 8/2
  Logical Operator12/1 -> Logical Operator24/2
  Logical Operator11/1 -> Logical Operator23/2
  Logical Operator22/1 -> Logical Operator25/1, 8/1
  Logical Operator21/1 -> Logical Operator24/1, 6/1
  Logical Operator20/1 -> Logical Operator23/1, 7/1
  Logical Operator/1 -> Logical Operator22/2, Logical Operator21/2, Logical Operator20/2
  Logical Operator19/1 -> Logical Operator22/1
  Logical Operator17/1 -> Logical Operator21/1
  Logical Operator15/1 -> Logical Operator20/1
  block_a/1 -> Logical Operator14/1
  block_b/1 -> Logical Operator16/1
  block_c/1 -> Logical Operator18/1
  5/1 -> Logical Operator19/1
  Logical Operator18/1 -> Logical Operator19/2
  3/1 -> Logical Operator17/1
  Logical Operator16/1 -> Logical Operator17/2
  4/1 -> Logical Operator15/1
  Logical Operator14/1 -> Logical Operator15/2
  Logical Operator10/1 -> Logical Operator13/2
  Logical Operator8/1 -> Logical Operator13/1
  Logical Operator7/1 -> Logical Operator12/2
  Logical Operator5/1 -> Logical Operator12/1
  Logical Operator4/1 -> Logical Operator11/2
  Logical Operator2/1 -> Logical Operator11/1
  Constant2/1 -> Logical Operator10/2, Logical Operator7/2, Logical Operator4/2
  dir_to_line_c/1 -> Logical Operator9/1, Logical Operator8/2
  dir_to_line_b/1 -> Logical Operator6/1, Logical Operator5/2
  Logical Operator9/1 -> Logical Operator10/1
  Logical Operator6/1 -> Logical Operator7/1
  Logical Operator3/1 -> Logical Operator4/1
  dir_to_line_a/1 -> Logical Operator3/1, Logical Operator2/2
  Constant1/1 -> Logical Operator5/1, Logical Operator8/1, Logical Operator2/1
  Relational Operator1/1 -> 4/1
  Constant3/1 -> Relational Operator4/2, Relational Operator5/2, Relational Operator3/2, Relational Operator/2, Relational Operator1/2, Relational Operator2/2
  Relational Operator3/1 -> 3/1
  Relational Operator5/1 -> 5/1
  Relational Operator4/1 -> 5/3
  Relational Operator2/1 -> 3/3
  Relational Operator/1 -> 4/3
  Constant/1 -> 4/2, 3/2, 5/2
  in_c_re/1 -> ORTOTOMODULE2/1
  in_c_im/1 -> ORTOTOMODULE2/2
  ORTOTOMODULE2/1 -> Relational Operator4/1, Relational Operator5/1
  in_b_im/1 -> ORTOTOMODULE1/2
  ORTOTOMODULE1/1 -> Relational Operator3/1, Relational Operator2/1
  ORTOTOMODULE/1 -> Relational Operator/1, Relational Operator1/1
  in_a_re/1 -> ORTOTOMODULE/1
  in_a_im/1 -> ORTOTOMODULE/2
  33/1 -> Logical Operator/1
  1/1 -> Logical Operator1/1
  Logical Operator1/1 -> Logical Operator/2
  no_dir4/1 -> 2/4
  no_dir3/1 -> 2/3
  no_dir2/1 -> 2/2
  no_dir1/1 -> 2/1
  block4/1 -> 1/4
  block3/1 -> 1/3
  block2/1 -> 1/2
  block1/1 -> 1/1
  start2/1 -> 33/2
  start3/1 -> 33/3
  start4/1 -> 33/4
  start1/1 -> 33/1

== system mylib/262_tnznp_line_st_v1/218_det18 ==
  start1 : Inport
  start2 : Inport  Port=2
  start3 : Inport  Port=3
  start4 : Inport  Port=4
  block1 : Inport  Port=5
  block2 : Inport  Port=6
  block3 : Inport  Port=7
  block4 : Inport  Port=8
  no_dir1 : Inport  Port=9
  no_dir2 : Inport  Port=10
  no_dir3 : Inport  Port=11
  no_dir4 : Inport  Port=12
  in_re : Inport  Port=13
  in_im : Inport  Port=14
  dir_to_line : Inport  Port=15
  1 : Logic  Operator=OR  Inputs=4  AllPortsSameDT=off  OutDataTypeStr=boolean
  2 : Logic  Operator=OR  Inputs=4  AllPortsSameDT=off  OutDataTypeStr=boolean
  33 : Logic  Operator=OR  Inputs=4  AllPortsSameDT=off  OutDataTypeStr=boolean
  4 : Switch  Criteria=u2 > Threshold
  7 : Switch  Criteria=u2 > Threshold
  Constant : Constant  Value=max_min
  Constant1 : Constant  Value=dir_to_line
  Constant2 : Constant  Value=dir_to_bus
  Constant3 : Constant  Value=set
  Logical Operator{,2,4,20,23} (5 alike) : Logic  AllPortsSameDT=off  OutDataTypeStr=boolean
  Logical Operator1 : Logic  Operator=NOT  AllPortsSameDT=off  OutDataTypeStr=boolean
  Logical Operator11 : Logic  Operator=OR  AllPortsSameDT=off  OutDataTypeStr=boolean
  Logical Operator3 : Logic  Operator=NOT  AllPortsSameDT=off  OutDataTypeStr=boolean
  ORTOTOMODULE : $bdroot/ORTOTOMODULE  SystemSampleTime=-1  Latency=0  AutoFrameSizeCalculation=off
  R_TRIG : $bdroot/R_TRIG  SystemSampleTime=-1  Latency=0  AutoFrameSizeCalculation=off
  Relational Operator : RelationalOperator  Operator=>  OutDataTypeStr=boolean  RndMeth=Simplest
  Relational Operator1 : RelationalOperator  Operator=<  OutDataTypeStr=boolean  RndMeth=Simplest
  avar : Outport
  Y : Outport  Port=2
  wires:
  R_TRIG/1 -> avar/1
  7/1 -> R_TRIG/1, Y/1
  Logical Operator23/1 -> 7/3
  2/1 -> 7/2
  Logical Operator11/1 -> Logical Operator23/2
  Logical Operator20/1 -> Logical Operator23/1, 7/1
  Logical Operator/1 -> Logical Operator20/2
  4/1 -> Logical Operator20/1
  Logical Operator4/1 -> Logical Operator11/2
  Logical Operator2/1 -> Logical Operator11/1
  Constant2/1 -> Logical Operator4/1
  Logical Operator3/1 -> Logical Operator4/2
  dir_to_line/1 -> Logical Operator3/1, Logical Operator2/2
  Constant1/1 -> Logical Operator2/1
  Relational Operator1/1 -> 4/1
  Constant3/1 -> Relational Operator/2, Relational Operator1/2
  Relational Operator/1 -> 4/3
  Constant/1 -> 4/2
  ORTOTOMODULE/1 -> Relational Operator/1, Relational Operator1/1
  in_re/1 -> ORTOTOMODULE/1
  in_im/1 -> ORTOTOMODULE/2
  33/1 -> Logical Operator/1
  1/1 -> Logical Operator1/1
  Logical Operator1/1 -> Logical Operator/2
  no_dir4/1 -> 2/4
  no_dir3/1 -> 2/3
  no_dir2/1 -> 2/2
  no_dir1/1 -> 2/1
  block4/1 -> 1/4
  block3/1 -> 1/3
  block2/1 -> 1/2
  block1/1 -> 1/1
  start2/1 -> 33/2
  start3/1 -> 33/3
  start4/1 -> 33/4
  start1/1 -> 33/1

== system mylib/262_tnznp_line_st_v1/230_st18_ph ==
  fast1_time : Inport
  fast2_time : Inport  Port=2
  fast1_zero : Inport  Port=3
  fast2_zero : Inport  Port=4
  block1 : Inport  Port=5
  block2 : Inport  Port=6
  block3 : Inport  Port=7
  block4 : Inport  Port=8
  in_a : Inport  Port=9
  in_b : Inport  Port=10
  in_c : Inport  Port=11
  alt_in_a : Inport  Port=12
  alt_in_b : Inport  Port=13
  alt_in_c : Inport  Port=14
  jmp_a : Inport  Port=15
  jmp_b : Inport  Port=16
  jmp_c : Inport  Port=17
  1 : Logic  Operator=OR  Inputs=4  AllPortsSameDT=off  OutDataTypeStr=boolean
  Constant1 : Constant  Value=only_K2
  Constant2 : Constant  Value=only_K3
  Constant3 : Constant  Value=only_K1
  Constant4 : Constant  Value=jmp_in_zone
  Logical Operator1 : Logic  Operator=OR  Inputs=3  AllPortsSameDT=off  OutDataTypeStr=boolean
  Logical Operator10 : Logic  Inputs=3  AllPortsSameDT=off  OutDataTypeStr=boolean
  Logical Operator{2,4,6,11..13} (6 alike) : Logic  AllPortsSameDT=off  OutDataTypeStr=boolean
  Logical Operator{14,16..17,27..28} (5 alike) : Logic  Operator=OR  AllPortsSameDT=off  OutDataTypeStr=boolean
  Logical Operator26 : Logic  Operator=OR  Inputs=3  AllPortsSameDT=off  OutDataTypeStr=boolean
  Logical Operator3 : Logic  Operator=NOT  AllPortsSameDT=off  OutDataTypeStr=boolean
  Logical Operator5 : Logic  Operator=NOT  AllPortsSameDT=off  OutDataTypeStr=boolean
  Logical Operator7 : Logic  Operator=NOT  AllPortsSameDT=off  OutDataTypeStr=boolean
  Logical Operator8 : Logic  Inputs=3  AllPortsSameDT=off  OutDataTypeStr=boolean
  Logical Operator9 : Logic  Inputs=3  AllPortsSameDT=off  OutDataTypeStr=boolean
  R_TRIG : $bdroot/R_TRIG  SystemSampleTime=-1  Latency=0  AutoFrameSizeCalculation=off
  Subsystem : Subsystem  mask{time=[T_fast, T_st]}
      mask prompts: time "time [T_fast, T_st]"
  in_1 : Subsystem  mask{in_jmp=[T_reset]}
      mask prompts: in_jmp "in_jmp[T_reset]"
  in_2 : Subsystem  mask{in_jmp=[T_reset]}
      mask prompts: in_jmp "in_jmp[T_reset]"
  in_3 : Subsystem  mask{in_jmp=[T_reset]}
      mask prompts: in_jmp "in_jmp[T_reset]"
  k_type : Subsystem
  out_a : $bdroot/out3  out=[T_out]
  out_b : $bdroot/out3  out=[T_out]
  out_c : $bdroot/out3  out=[T_out]
  avar : Outport
  Y : Outport  Port=2
  Y_a : Outport  Port=3
  Y_b : Outport  Port=4
  Y_c : Outport  Port=5
  fast : Outport  Port=6
  fast_a : Outport  Port=7
  fast_b : Outport  Port=8
  fast_c : Outport  Port=9
  wires:
  Logical Operator1/1 -> fast/1
  Logical Operator28/1 -> Subsystem/2(T_fast_zero)
  Logical Operator27/1 -> Subsystem/1(T_fast_time)
  alt_in_c/1 -> Logical Operator17/2
  alt_in_b/1 -> Logical Operator16/2
  alt_in_a/1 -> Logical Operator14/2
  Logical Operator14/1 -> Subsystem/3("In1 ")
  Logical Operator16/1 -> Subsystem/4("In2 ")
  Logical Operator17/1 -> Subsystem/5("In3 ")
  Logical Operator13/1 -> Logical Operator17/1
  Logical Operator12/1 -> Logical Operator16/1
  Logical Operator11/1 -> Logical Operator14/1
  k_type/1(out) -> Logical Operator11/1, Logical Operator13/1, Logical Operator12/1, Logical Operator8/3, Logical Operator9/3, Logical Operator10/3
  Constant2/1 -> k_type/6(only_K3)
  Constant1/1 -> k_type/5(only_K2)
  Constant3/1 -> k_type/4(only_K1)
  Logical Operator6/1 -> k_type/3(In_ c), Logical Operator13/2, fast_c/1, Logical Operator1/3
  Logical Operator4/1 -> k_type/2(In_b), Logical Operator12/2, fast_b/1, Logical Operator1/2
  Logical Operator2/1 -> k_type/1(In_a), Logical Operator11/2, fast_a/1, Logical Operator1/1
  Subsystem/1(Out1) -> Logical Operator8/2
  Subsystem/2(Out2) -> Logical Operator9/2
  Subsystem/3(Out3) -> Logical Operator10/2
  Logical Operator10/1 -> out_c/1
  Logical Operator9/1 -> out_b/1
  Logical Operator8/1 -> out_a/1
  out_c/1 -> Y_c/1, Logical Operator26/3  "Y_c"
  out_b/1 -> Y_b/1, Logical Operator26/2  "Y_c"
  out_a/1 -> Y_a/1, Logical Operator26/1  "Y_c"
  1/1 -> Logical Operator3/1, Logical Operator5/1, Logical Operator7/1
  in_3/1(Y) -> Logical Operator6/2  "Yc"
  Logical Operator7/1 -> Logical Operator6/1
  in_2/1(Y) -> Logical Operator4/2  "Yb"
  Logical Operator5/1 -> Logical Operator4/1
  in_1/1(Y) -> Logical Operator2/2  "Ya"
  Logical Operator3/1 -> Logical Operator2/1
  jmp_c/1 -> in_3/3(jmp)
  jmp_b/1 -> in_2/3(jmp)
  jmp_a/1 -> in_1/3(jmp)
  Constant4/1 -> in_1/1(jmp_in_zone), in_2/1(jmp_in_zone), in_3/1(jmp_in_zone)
  in_b/1 -> Logical Operator9/1, in_2/2(in)
  R_TRIG/1 -> avar/1
  Logical Operator26/1 -> R_TRIG/1, Y/1
  in_c/1 -> Logical Operator10/1, in_3/2(in)
  in_a/1 -> Logical Operator8/1, in_1/2(in)
  block4/1 -> 1/4
  block3/1 -> 1/3
  block2/1 -> 1/2
  block1/1 -> 1/1
  fast2_time/1 -> Logical Operator27/2
  fast1_zero/1 -> Logical Operator28/1
  fast2_zero/1 -> Logical Operator28/2
  fast1_time/1 -> Logical Operator27/1
